simulink model "rlwatertank"  (R2022b)
settings: Solver=ode45  StartTime=0.0  StopTime=inf  RelTol=1e-3  EnableMultiTasking=on
PreLoadFcn:
  | watertankdat
model workspace (MAT data in the model file):
  deltaref = 1
  prevref = 0
undefined symbols (not defined in the file): a, A, b, DiscIntNeverNeededParam, random_refs_table, Ts
libraries: simulink x3, rllib x1
settings Model: Creator=The MathWorks, Inc.  LastModifiedBy=enes
settings SolverCC: AlgebraicLoopSolver=TrustRegion
settings DataIOCC: LimitDataPoints=on  SaveFormat=Array  SignalLoggingName=logsOut
settings OptimizationCC: ExpressionDepthLimit=2147483647  InitFltsAndDblsToZero=on  LifeSpan=inf
settings DebuggingCC: SaveWithParameterizedLinksMsg=none  UnderspecifiedInitializationDetection=Classic  MergeDetectMultiDrivingBlocksExec=none  SignalResolutionControl=TryResolveAllWithWarning  MultiTaskDSMMsg=warning  FcnCallInpInsideContextMsg=warning  UnconnectedInputMsg=warning  UnconnectedOutputMsg=warning  UnconnectedLineMsg=warning  AllowSymbolicDim=off  StateNameClashWarn=warning  SFUnexpectedBacktrackingDiag=warning  SFNoUnconditionalDefaultTransitionDiag=warning  SFExecutionAtInitializationDiag=none  SFMachineParentedDataDiag=warning  ArithmeticOperatorsInVariantConditions=warning
settings HardwareCC: ProdBitPerPointer=32  ProdBitPerSizeT=32  ProdBitPerPtrDiffT=32  ProdLargestAtomicFloat=None  ProdIntDivRoundTo=Undefined  ProdEndianess=Unspecified  ProdWordSize=32  ProdHWDeviceType=Specified
settings ModelReferenceCC: EnableRefExpFcnMdlSchedulingChecks=on  PropagateSignalLabelsOutOfModel=off
settings SFSimCC: SimUseLocalCustomCode=off  CustomCodeUndefinedFunction=UseInterfaceOnly
settings RTWCC: RTWUseLocalCustomCode=off
settings CodeAppCC: StateflowObjectComments=on
settings GRTTargetCC: TargetFcnLib=ansi_tfl_tmw.mat  TargetLangStandard=C89/C90 (ANSI)  CombineOutputUpdateFcns=off  GRTInterface=on
settings ConfigComp: CovMetricSettings=dw  CovSaveCumulativeToWorkspaceVar=on  CovSaveSingleToWorkspaceVar=on  CovExternalEMLEnable=off

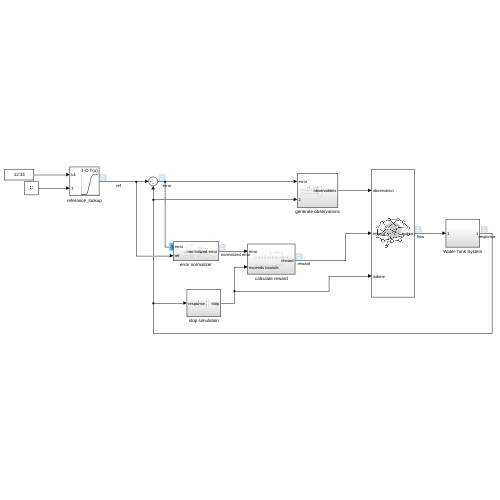
[thumbnail: Simulink's stored preview of the top-level diagram]
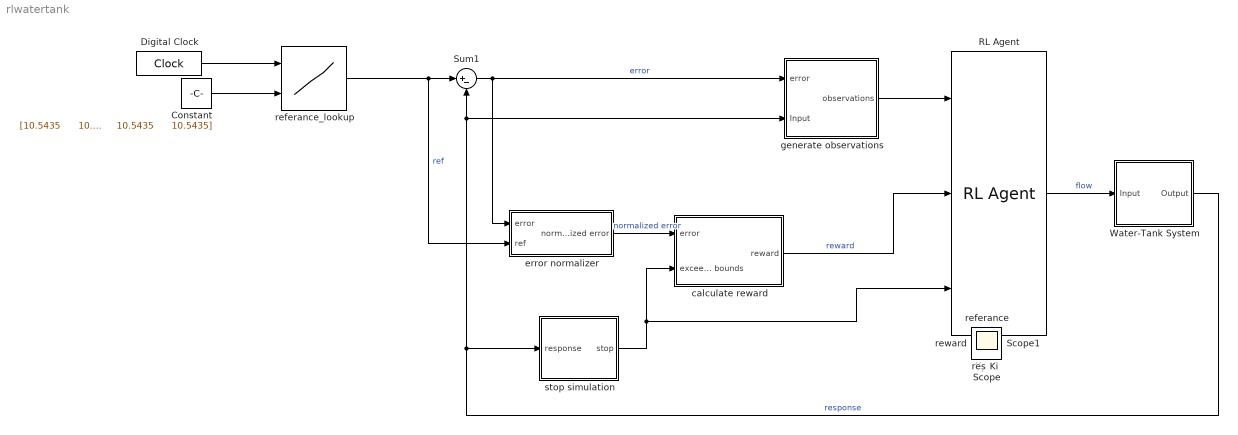
== system rlwatertank ==
  Constant : Constant  Value="[10.5435      10.5435      10.5435      10.5435      10.5435      10.5435      10.5435      10.5435      10.5435      10.5435      10.5435      10.5435      10.5435      10.5435      10.5435      10.5435      10.5435      10.5435      10.5435      10.5435      10.5435      10.5435      10.5435      10.5435      10.5435      10.5435      10.5435      10.5435      10.5435      10.5435      10.5435      10.5435      10.5435      10.5435      10.5435      10.5435      10.5435      10.5435      10.5435      10.5435      10.5435      10.5435      10.5435      10.5435      10.5435      10.5435      10.5435      10.5435      10.5435      10.5435      10.5435      10.5435      10.5435      10.5435      10.5435      10.5435      10.5435      10.5435      10.5435      10.5435      10.5435      10.5435      10.5435      10.5435      10.5435      10.5435      10.5435      10.5435      10.5435      10.5435      10.5435      10.5435      10.5435      10.5435      10.5435      10.5435      10.5435      10.5435      10.5435      10.5435      10.5435      10.5435      10.5435      10.5435      10.5435      10.5435      10.5435      10.5435      10.5435      10.5435      10.5435      10.5435      10.5435      10.5435      10.5435      10.5435      10.5435      10.5435      10.5435      10.5435      10.5435      10.5435      10.5435      10.5435      10.5435      10.5435      10.5435      10.5435      10.5435      10.5435      10.5435      10.5435      10.5435      10.5435      10.5435      10.5435      10.5435      10.5435      10.5435      10.5435      10.5435      10.5435      10.5435      10.5435      10.5435      10.5435      10.5435      10.5435      10.5435      10.5435      10.5435      10.5435      10.5435      10.5435      10.5435      10.5435      10.5435      10.5435      10.5435      10.5435      10.5435      10.5435      10.5435      10.5435      10.5435      10.5435      10.5435      10.5435      10.5435      10.5435      10.5435      10.5435      10.5435      10.5435      10.5435      10.5435      10.5435      10.5435      10.5435      10.5435      10.5435      10.5435      10.5435      10.5435      10.5435      10.5435      10.5435      10.5435      10.5435      10.5435      10.5435      10.5435      10.5435      10.5435      10.5435      10.5435      10.5435      10.5435      10.5435      10.5435      10.5435      10.5435      10.5435      10.5435      10.5435      10.5435      10.5435      10.5435      10.5435      10.5435      10.5435      10.5435      10.5435      10.5435      10.5435      10.5435      10.5435      10.5435      10.5435      10.5435]"
  Digital Clock : DigitalClock
  RL Agent : rllib/RL Agent  Agent=agent  ExternalActionAsInput=off  ProvideLastAction=off  ProvideCumRwd=off  TreatAsDirectFeedthrough=on  UseStrictObservationDataTypes=off
  Sum1 : Sum  Inputs=|+-  SaturateOnIntegerOverflow=on
  Water-Tank System : Subsystem
  calculate reward : Subsystem
  error normalizer : Subsystem
  generate observations : Subsystem
  referance_lookup : Lookup_n-D  NumberOfTableDimensions=1  BreakpointsForDimension1=[1:200]  TableSource=Input port  Table=random_refs_table  InternalRulePriority=Speed  RndMeth=Simplest
      settings: InputPortMap=u0,p221
  stop simulation : Subsystem
  Kp Ki : Scope
  Scope : Scope
  Scope1 : Scope
  error : Scope
  referance : Scope
  res : Scope
  reward : Scope
  wires:
  RL Agent/1 -> Water-Tank System/1(Input)  "flow"
  generate observations/1(observations) -> RL Agent/1
  calculate reward/1(reward) -> RL Agent/2  "reward"
  stop simulation/1(stop) -> calculate reward/2(exceeds bounds), RL Agent/3
  referance_lookup/1 -> error normalizer/2(ref), Sum1/1  "ref"
  Digital Clock/1 -> referance_lookup/1
  Sum1/1 -> error normalizer/1(error), generate observations/1(error)  "error"
  Water-Tank System/1(Output) -> stop simulation/1(response), Sum1/2, generate observations/2(Input)  "response"
  Constant/1 -> referance_lookup/2
  error normalizer/1(normalized error) -> calculate reward/1(error)  "normalized error"

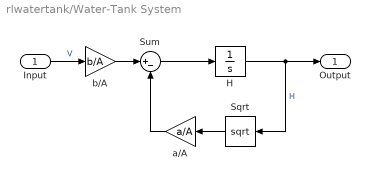
== system rlwatertank/Water-Tank System ==
  Input : Inport
  H : Integrator  InitialCondition=10.1628  LimitOutput=on  LowerSaturationLimit=0
  Sqrt : Sqrt  OutputSignalType=real
  Sum : Sum  Inputs=|+-  SaturateOnIntegerOverflow=on
  a/A : Gain  Gain=a/A  SaturateOnIntegerOverflow=on  OutDataTypeStr=Inherit: Same as input  ParamDataTypeStr=Inherit: Same as input
  b/A : Gain  Gain=b/A  SaturateOnIntegerOverflow=on  OutDataTypeStr=Inherit: Same as input  ParamDataTypeStr=Inherit: Same as input
  Output : Outport  VectorParamsAs1DForOutWhenUnconnected=off
  wires:
  b/A/1 -> Sum/1
  Sum/1 -> H/1
  H/1 -> Sqrt/1, Output/1  "H"
  Sqrt/1 -> a/A/1
  a/A/1 -> Sum/2
  Input/1 -> b/A/1  "V"

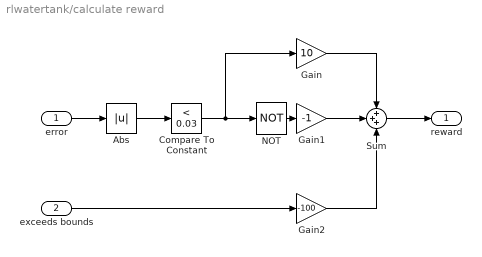
== system rlwatertank/calculate reward ==
  error : Inport
  exceeds bounds : Inport  Port=2
  Abs : Abs  SaturateOnIntegerOverflow=off
  Compare To Constant : simulink/Logic and Bit Operations/Compare To Constant  relop=<  const=0.03  OutDataTypeStr=boolean
  Gain : Gain  Gain=10
  Gain1 : Gain  Gain=-1
  Gain2 : Gain  Gain=-100
  NOT : Logic  Operator=NOT  IconShape=distinctive  AllPortsSameDT=off  OutDataTypeStr=boolean
  Sum : Sum  Inputs=+++  OutDataTypeStr=double
  reward : Outport  VectorParamsAs1DForOutWhenUnconnected=off
  wires:
  Abs/1 -> Compare To Constant/1
  Gain2/1 -> Sum/3
  Gain/1 -> Sum/1
  Compare To Constant/1 -> NOT/1, Gain/1
  Gain1/1 -> Sum/2
  Sum/1 -> reward/1
  NOT/1 -> Gain1/1
  exceeds bounds/1 -> Gain2/1
  error/1 -> Abs/1

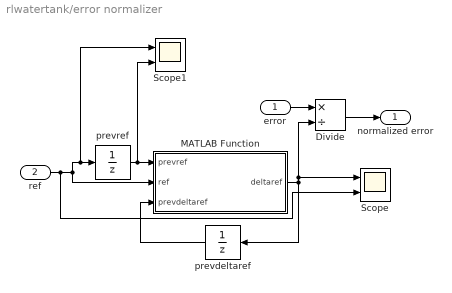
== system rlwatertank/error normalizer ==
  error : Inport
  ref : Inport  Port=2
  Divide : Product  Inputs=*/
  MATLAB Function : MATLAB Function  TreatAsAtomicUnit=on
  Scope : Scope  NumInputPorts=2
  Scope1 : Scope  NumInputPorts=2
  prevdeltaref : UnitDelay  SampleTime=-1  HasFrameUpgradeWarning=on
  prevref : UnitDelay  SampleTime=-1  HasFrameUpgradeWarning=on
  normalized error : Outport
  wires:
  prevdeltaref/1 -> MATLAB Function/3(prevdeltaref)
  MATLAB Function/1(deltaref) -> Scope/1, Divide/2, prevdeltaref/1
  prevref/1 -> Scope1/2, MATLAB Function/1(prevref)
  ref/1 -> Scope/2, Scope1/1, prevref/1, MATLAB Function/2(ref)
  error/1 -> Divide/1
  Divide/1 -> normalized error/1

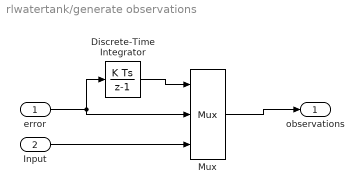
== system rlwatertank/generate observations ==
  error : Inport
  Input : Inport  Port=2
  Discrete-Time Integrator : DiscreteIntegrator  SampleTime=Ts  ICPrevOutput=DiscIntNeverNeededParam  ICPrevScaledInput=DiscIntNeverNeededParam
  Mux : Mux  Inputs=3
  observations : Outport  VectorParamsAs1DForOutWhenUnconnected=off
  wires:
  Discrete-Time Integrator/1 -> Mux/1
  error/1 -> Discrete-Time Integrator/1, Mux/2
  Mux/1 -> observations/1
  Input/1 -> Mux/3

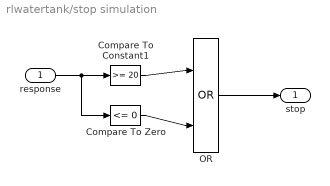
== system rlwatertank/stop simulation ==
  response : Inport
  Compare To Constant1 : simulink/Logic and Bit Operations/Compare To Constant  relop=>=  const=20  OutDataTypeStr=boolean
  Compare To Zero : simulink/Logic and Bit Operations/Compare To Zero  relop=<=  OutDataTypeStr=boolean
  OR : Logic  Operator=OR  IconShape=distinctive  AllPortsSameDT=off  OutDataTypeStr=boolean
  stop : Outport  VectorParamsAs1DForOutWhenUnconnected=off
  wires:
  response/1 -> Compare To Zero/1, Compare To Constant1/1
  Compare To Zero/1 -> OR/2
  Compare To Constant1/1 -> OR/1
  OR/1 -> stop/1

== matlab function rlwatertank/error normalizer/MATLAB Function ==
  data: prevref input; deltaref output; ref input; prevdeltaref input
function deltaref = fcn(prevref, ref,prevdeltaref)

delta = abs(prevref - ref);
if delta ~= 0
    deltaref = delta;
else
    deltaref = prevdeltaref;
end
